simulink subsystem "ElevationCheck"  (R2021a)
settings: Solver=VariableStepAuto  StartTime=0.0  StopTime=10.0  RelTol=1e-3
undefined symbols (not defined in the file): ErrCodeEl, NoErr, RangeLwEl, RangeUpEl
libraries: simulink x1
settings Model: Creator=zurnmar  LastModifiedBy=zurnmar

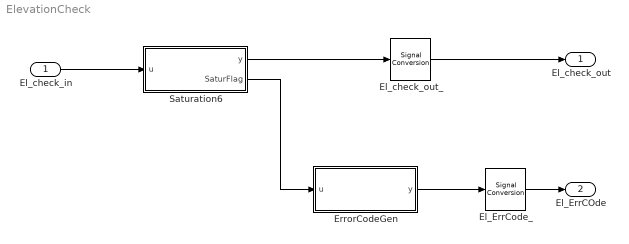
== system ElevationCheck ==
  El_check_in : Inport
  El_ErrCode_ : SignalConversion  OverrideOpt=off
  El_check_out_ : SignalConversion  OverrideOpt=off
  ErrorCodeGen : Subsystem
  Saturation6 : Subsystem  TreatAsAtomicUnit=on
      settings: RTWFcnNameOpts=Use subsystem name
  El_check_out : Outport
  El_ErrCOde : Outport  Port=2
  wires:
  ErrorCodeGen/1(y) -> El_ErrCode_/1
  El_check_in/1 -> Saturation6/1(u)
  Saturation6/1(y) -> El_check_out_/1
  Saturation6/2(SaturFlag) -> ErrorCodeGen/1(u)
  El_check_out_/1 -> El_check_out/1
  El_ErrCode_/1 -> El_ErrCOde/1

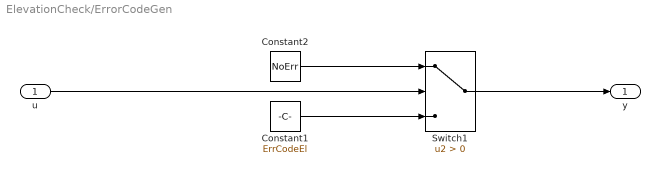
== system ElevationCheck/ErrorCodeGen ==
  u : Inport
  Constant1 : Constant  Value=ErrCodeEl  OutDataTypeStr=uint16
  Constant2 : Constant  Value=NoErr
  Switch1 : Switch  Criteria=u2 > Threshold
  y : Outport
  wires:
  Switch1/1 -> y/1
  Constant1/1 -> Switch1/3
  Constant2/1 -> Switch1/1
  u/1 -> Switch1/2

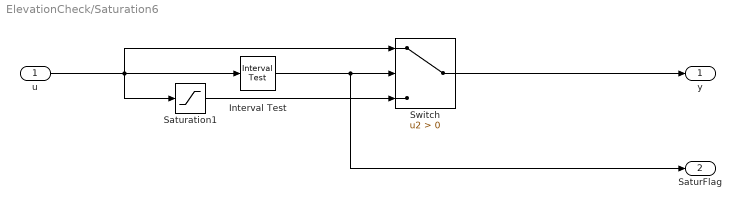
== system ElevationCheck/Saturation6 ==
  u : Inport
  Interval Test : simulink/Logic and Bit Operations/Interval Test  IntervalClosedRight=on  uplimit=RangeUpEl  IntervalClosedLeft=on  lowlimit=RangeLwEl  OutDataTypeStr=boolean
  Saturation1 : Saturate  UpperLimit=RangeUpEl  LowerLimit=RangeLwEl
  Switch : Switch  Criteria=u2 > Threshold
  y : Outport
  SaturFlag : Outport  Port=2
  wires:
  Saturation1/1 -> Switch/3
  Switch/1 -> y/1
  u/1 -> Interval Test/1, Switch/1, Saturation1/1
  Interval Test/1 -> Switch/2, SaturFlag/1
